simulink model "compare_model"  (R2022b)
settings: Solver=VariableStepAuto  StartTime=0.0  StopTime=t_samples*n_samples  RelTol=1e-3
values from neighbouring files (symbols this model uses):
  air_den = 1.225    [wind_turbine_parameters.m]
  l1 = 56    [wind_turbine_parameters.m]
  lambda_op = 5.68    [wind_turbine_parameters.m]
undefined symbols (not defined in the file or in its folder): pitch_deg, t_sample2
libraries: simulink x1, fuzblock x1
settings Model: Creator=luan  LastModifiedBy=marina

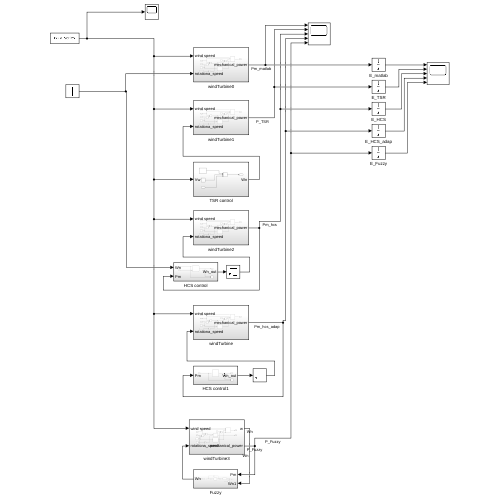
[thumbnail: Simulink's stored preview of the top-level diagram]
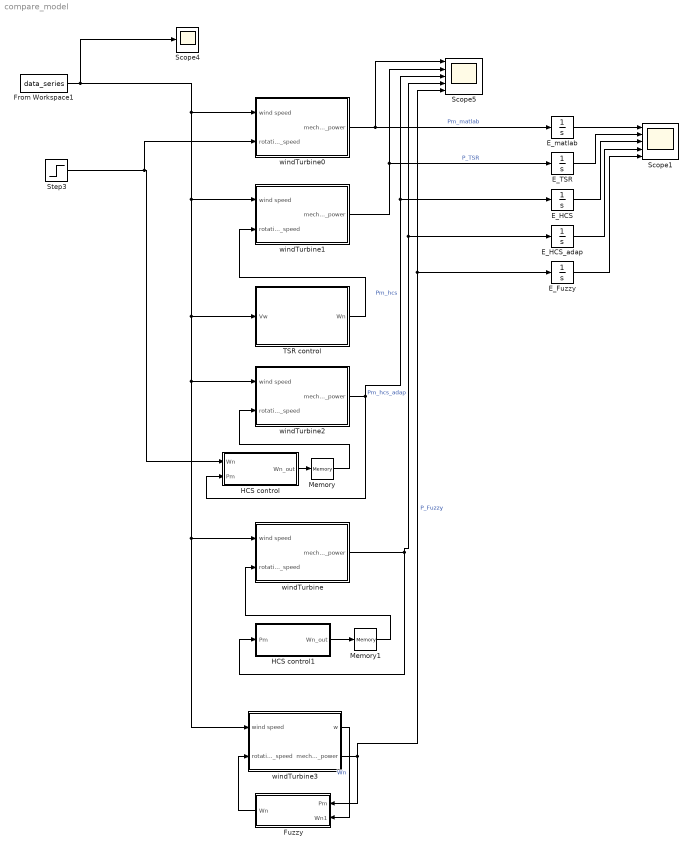
== system compare_model ==
  E_Fuzzy : Integrator
  E_HCS : Integrator
  E_HCS_adap : Integrator
  E_TSR : Integrator
  E_matlab : Integrator
  From Workspace1 : FromWorkspace  VariableName=data_series  SampleTime=t_sample2  OutputAfterFinalValue=Setting to zero
  Fuzzy : Subsystem
  HCS control : Subsystem
  HCS control1 : Subsystem
  Memory : Memory
  Memory1 : Memory
  Scope1 : Scope  NumInputPorts=5
  Scope4 : Scope
  Scope5 : Scope  NumInputPorts=5
  Step3 : Step  Time=0  After=0.9  SampleTime=0
  TSR control : Subsystem
  windTurbine : Subsystem
  windTurbine0 : Subsystem
  windTurbine1 : Subsystem
  windTurbine2 : Subsystem
  windTurbine3 : Subsystem
  wires:
  windTurbine0/1(mechanical_power) -> Scope5/1, E_matlab/1  "Pm_matlab"
  E_matlab/1 -> Scope1/1
  From Workspace1/1 -> Scope4/1, windTurbine0/1(wind speed), windTurbine1/1(wind speed), windTurbine2/1(wind speed), windTurbine3/1(wind speed), windTurbine/1(wind speed), TSR control/1(Vw)
  Step3/1 -> windTurbine0/2(rotationa_speed), HCS control/1(Wn)
  TSR control/1(Wn) -> windTurbine1/2(rotationa_speed)
  HCS control/1(Wn_out) -> Memory/1
  windTurbine2/1(mechanical_power) -> E_HCS/1, Scope5/3, HCS control/2(Pm)  "Pm_hcs"
  windTurbine/1(mechanical_power) -> E_HCS_adap/1, Scope5/4, HCS control1/1(Pm)  "Pm_hcs_adap"
  HCS control1/1(Wn_out) -> Memory1/1
  Memory1/1 -> windTurbine/2(rotationa_speed)
  windTurbine3/2(mechanical_power) -> E_Fuzzy/1, Scope5/5, Fuzzy/1(Pm)  "P_Fuzzy"
  windTurbine3/1(w) -> Fuzzy/2(Wn1)  "Wn"
  windTurbine1/1(mechanical_power) -> E_TSR/1, Scope5/2  "P_TSR"
  E_TSR/1 -> Scope1/2
  E_HCS_adap/1 -> Scope1/4
  E_HCS/1 -> Scope1/3
  E_Fuzzy/1 -> Scope1/5
  Memory/1 -> windTurbine2/2(rotationa_speed)
  Fuzzy/1(Wn) -> windTurbine3/2(rotationa_speed)

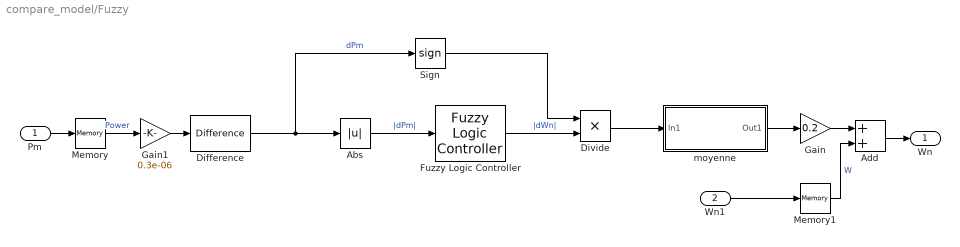
== system compare_model/Fuzzy ==
  Pm : Inport
  Wn1 : Inport  Port=2
  Abs : Abs  SaturateOnIntegerOverflow=off
  Add : Sum
  Difference : simulink/Discrete/Difference  ICPrevInput=0.0  OutMin=[]  OutMax=[]  OutDataType=fixdt(1, 16)  OutScaling=2^-10  DoSatur=off
  Divide : Product  Inputs=**
  Fuzzy Logic Controller : fuzblock/Fuzzy Logic  Controller  FIS='version1.fis'  OutputSampleNumber=101  DataType=double  FuzzifiedInputs=off  RuleFiringStrengths=off  RuleOutputs=off  AggregatedOutputs=off  SimulateUsing=Interpreted execution  OutOfRangeInputValueMessage=warning  NoRuleFiredMessage=warning  EmptyOutputFuzzySetMessage=warning
  Gain : Gain  Gain=0.2
  Gain1 : Gain  Gain=0.3e-06
  Memory : Memory
  Memory1 : Memory  InitialCondition=0.2
  Sign : Signum
  moyenne : Subsystem
  Wn : Outport
  wires:
  Abs/1 -> Fuzzy Logic Controller/1  "|dPm|"
  Add/1 -> Wn/1
  Difference/1 -> Sign/1, Abs/1  "dPm"
  Sign/1 -> Divide/1
  Fuzzy Logic Controller/1 -> Divide/2  "|dWn|"
  Divide/1 -> moyenne/1(In1)
  moyenne/1(Out1) -> Gain/1
  Gain/1 -> Add/1
  Gain1/1 -> Difference/1
  Memory1/1 -> Add/2  "W"
  Memory/1 -> Gain1/1  "Power"
  Pm/1 -> Memory/1
  Wn1/1 -> Memory1/1

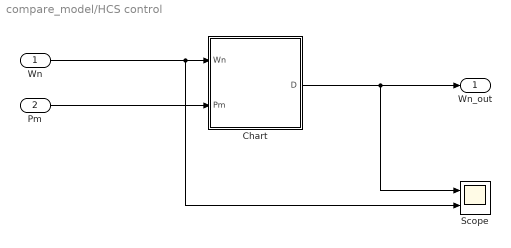
== system compare_model/HCS control ==
  Wn : Inport
  Pm : Inport  Port=2
  Chart : Stateflow chart  TreatAsAtomicUnit=on
  Scope : Scope  NumInputPorts=2
  Wn_out : Outport
  wires:
  Pm/1 -> Chart/2(Pm)
  Wn/1 -> Scope/2, Chart/1(Wn)
  Chart/1(D) -> Scope/1, Wn_out/1

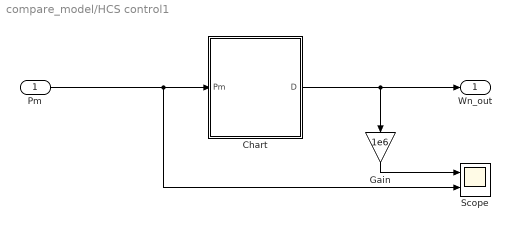
== system compare_model/HCS control1 ==
  Pm : Inport
  Chart : Stateflow chart  TreatAsAtomicUnit=on
  Gain : Gain  Gain=1e6
  Scope : Scope  NumInputPorts=2
  Wn_out : Outport
  wires:
  Chart/1(D) -> Gain/1, Wn_out/1
  Pm/1 -> Scope/2, Chart/1(Pm)
  Gain/1 -> Scope/1

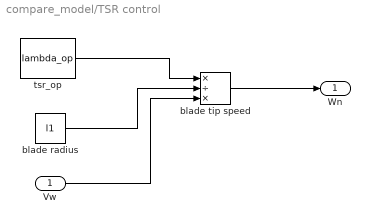
== system compare_model/TSR control ==
  Vw : Inport
  blade radius : Constant  Value=l1
  blade tip speed : Product  Inputs=*/*
  tsr_op : Constant  Value=lambda_op
  Wn : Outport
  wires:
  blade tip speed/1 -> Wn/1
  Vw/1 -> blade tip speed/3
  tsr_op/1 -> blade tip speed/1
  blade radius/1 -> blade tip speed/2

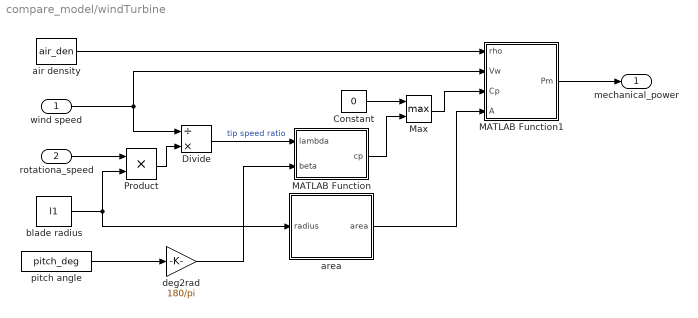
== system compare_model/windTurbine ==
  wind speed : Inport
  rotationa_speed : Inport  Port=2
  Constant : Constant  Value=0
  Divide : Product  Inputs=/*
  MATLAB Function : MATLAB Function  TreatAsAtomicUnit=on
  MATLAB Function1 : MATLAB Function  TreatAsAtomicUnit=on
  Max : MinMax  Function=max  Inputs=2
  Product : Product
  air density : Constant  Value=air_den
  area : Subsystem
  blade radius : Constant  Value=l1
  deg2rad : Gain  Gain=180/pi
  pitch angle : Constant  Value=pitch_deg
  mechanical_power : Outport
  wires:
  Product/1 -> Divide/2
  wind speed/1 -> Divide/1, MATLAB Function1/2(Vw)
  Divide/1 -> MATLAB Function/1(lambda)  "tip speed ratio"
  MATLAB Function1/1(Pm) -> mechanical_power/1
  rotationa_speed/1 -> Product/1
  air density/1 -> MATLAB Function1/1(rho)
  area/1(area) -> MATLAB Function1/4(A)
  blade radius/1 -> Product/2, area/1(radius)
  deg2rad/1 -> MATLAB Function/2(beta)
  Max/1 -> MATLAB Function1/3(Cp)
  MATLAB Function/1(cp) -> Max/2
  Constant/1 -> Max/1
  pitch angle/1 -> deg2rad/1

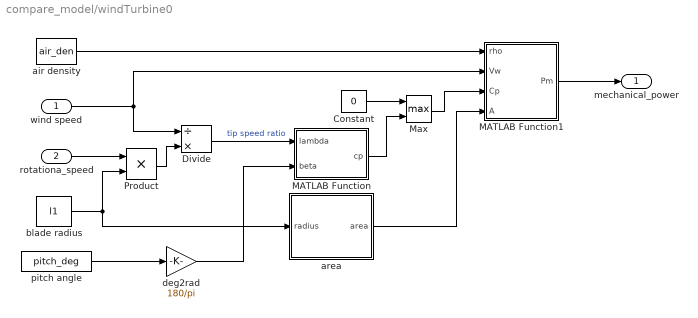
== system compare_model/windTurbine0 ==
  wind speed : Inport
  rotationa_speed : Inport  Port=2
  Constant : Constant  Value=0
  Divide : Product  Inputs=/*
  MATLAB Function : MATLAB Function  TreatAsAtomicUnit=on
  MATLAB Function1 : MATLAB Function  TreatAsAtomicUnit=on
  Max : MinMax  Function=max  Inputs=2
  Product : Product
  air density : Constant  Value=air_den
  area : Subsystem
  blade radius : Constant  Value=l1
  deg2rad : Gain  Gain=180/pi
  pitch angle : Constant  Value=pitch_deg
  mechanical_power : Outport
  wires:
  Product/1 -> Divide/2
  wind speed/1 -> Divide/1, MATLAB Function1/2(Vw)
  Divide/1 -> MATLAB Function/1(lambda)  "tip speed ratio"
  MATLAB Function1/1(Pm) -> mechanical_power/1
  rotationa_speed/1 -> Product/1
  air density/1 -> MATLAB Function1/1(rho)
  area/1(area) -> MATLAB Function1/4(A)
  blade radius/1 -> Product/2, area/1(radius)
  deg2rad/1 -> MATLAB Function/2(beta)
  Max/1 -> MATLAB Function1/3(Cp)
  MATLAB Function/1(cp) -> Max/2
  Constant/1 -> Max/1
  pitch angle/1 -> deg2rad/1

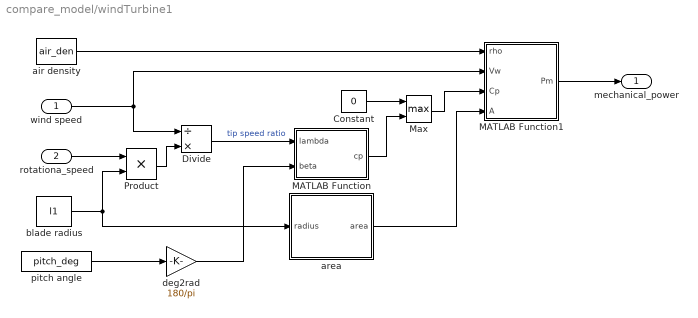
== system compare_model/windTurbine1 ==
  wind speed : Inport
  rotationa_speed : Inport  Port=2
  Constant : Constant  Value=0
  Divide : Product  Inputs=/*
  MATLAB Function : MATLAB Function  TreatAsAtomicUnit=on
  MATLAB Function1 : MATLAB Function  TreatAsAtomicUnit=on
  Max : MinMax  Function=max  Inputs=2
  Product : Product
  air density : Constant  Value=air_den
  area : Subsystem
  blade radius : Constant  Value=l1
  deg2rad : Gain  Gain=180/pi
  pitch angle : Constant  Value=pitch_deg
  mechanical_power : Outport
  wires:
  Product/1 -> Divide/2
  wind speed/1 -> Divide/1, MATLAB Function1/2(Vw)
  Divide/1 -> MATLAB Function/1(lambda)  "tip speed ratio"
  MATLAB Function1/1(Pm) -> mechanical_power/1
  rotationa_speed/1 -> Product/1
  air density/1 -> MATLAB Function1/1(rho)
  area/1(area) -> MATLAB Function1/4(A)
  blade radius/1 -> Product/2, area/1(radius)
  deg2rad/1 -> MATLAB Function/2(beta)
  Max/1 -> MATLAB Function1/3(Cp)
  MATLAB Function/1(cp) -> Max/2
  Constant/1 -> Max/1
  pitch angle/1 -> deg2rad/1

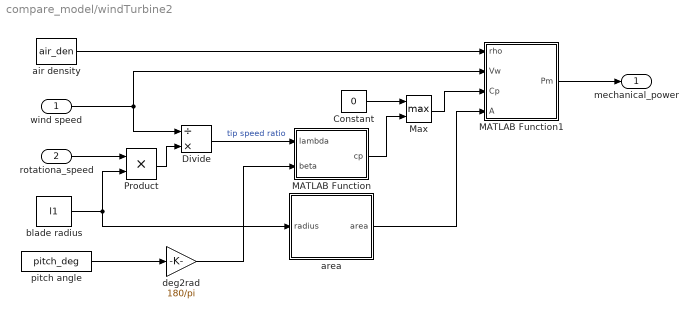
== system compare_model/windTurbine2 ==
  wind speed : Inport
  rotationa_speed : Inport  Port=2
  Constant : Constant  Value=0
  Divide : Product  Inputs=/*
  MATLAB Function : MATLAB Function  TreatAsAtomicUnit=on
  MATLAB Function1 : MATLAB Function  TreatAsAtomicUnit=on
  Max : MinMax  Function=max  Inputs=2
  Product : Product
  air density : Constant  Value=air_den
  area : Subsystem
  blade radius : Constant  Value=l1
  deg2rad : Gain  Gain=180/pi
  pitch angle : Constant  Value=pitch_deg
  mechanical_power : Outport
  wires:
  Product/1 -> Divide/2
  wind speed/1 -> Divide/1, MATLAB Function1/2(Vw)
  Divide/1 -> MATLAB Function/1(lambda)  "tip speed ratio"
  MATLAB Function1/1(Pm) -> mechanical_power/1
  rotationa_speed/1 -> Product/1
  air density/1 -> MATLAB Function1/1(rho)
  area/1(area) -> MATLAB Function1/4(A)
  blade radius/1 -> Product/2, area/1(radius)
  deg2rad/1 -> MATLAB Function/2(beta)
  Max/1 -> MATLAB Function1/3(Cp)
  MATLAB Function/1(cp) -> Max/2
  Constant/1 -> Max/1
  pitch angle/1 -> deg2rad/1

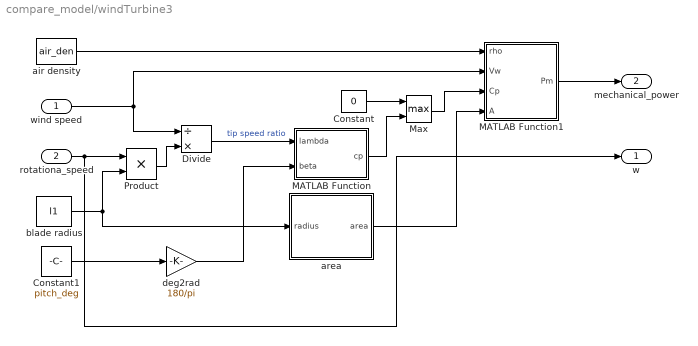
== system compare_model/windTurbine3 ==
  wind speed : Inport
  rotationa_speed : Inport  Port=2
  Constant : Constant  Value=0
  Constant1 : Constant  Value=pitch_deg
  Divide : Product  Inputs=/*
  MATLAB Function : MATLAB Function  TreatAsAtomicUnit=on
  MATLAB Function1 : MATLAB Function  TreatAsAtomicUnit=on
  Max : MinMax  Function=max  Inputs=2
  Product : Product
  air density : Constant  Value=air_den
  area : Subsystem
  blade radius : Constant  Value=l1
  deg2rad : Gain  Gain=180/pi
  w : Outport
  mechanical_power : Outport  Port=2
  wires:
  Product/1 -> Divide/2
  wind speed/1 -> Divide/1, MATLAB Function1/2(Vw)
  Divide/1 -> MATLAB Function/1(lambda)  "tip speed ratio"
  Constant1/1 -> deg2rad/1
  MATLAB Function1/1(Pm) -> mechanical_power/1
  rotationa_speed/1 -> w/1, Product/1
  air density/1 -> MATLAB Function1/1(rho)
  area/1(area) -> MATLAB Function1/4(A)
  blade radius/1 -> Product/2, area/1(radius)
  deg2rad/1 -> MATLAB Function/2(beta)
  Max/1 -> MATLAB Function1/3(Cp)
  MATLAB Function/1(cp) -> Max/2
  Constant/1 -> Max/1

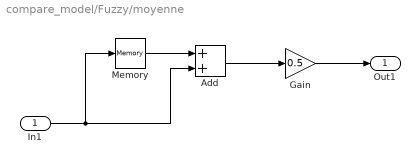
== system compare_model/Fuzzy/moyenne ==
  In1 : Inport
  Add : Sum
  Gain : Gain  Gain=0.5
  Memory : Memory
  Out1 : Outport
  wires:
  In1/1 -> Memory/1, Add/2
  Memory/1 -> Add/1
  Add/1 -> Gain/1
  Gain/1 -> Out1/1

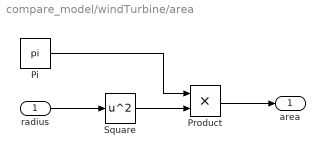
== system compare_model/windTurbine/area ==
  radius : Inport
  Pi : Constant  Value=pi  OutDataTypeStr=Inherit: Inherit via back propagation
  Product : Product
  Square : Math  Operator=square
  area : Outport
  wires:
  radius/1 -> Square/1
  Square/1 -> Product/2
  Pi/1 -> Product/1
  Product/1 -> area/1

== system compare_model/windTurbine0/area ==
  radius : Inport
  Pi : Constant  Value=pi  OutDataTypeStr=Inherit: Inherit via back propagation
  Product : Product
  Square : Math  Operator=square
  area : Outport
  wires:
  radius/1 -> Square/1
  Square/1 -> Product/2
  Pi/1 -> Product/1
  Product/1 -> area/1

== system compare_model/windTurbine1/area ==
  radius : Inport
  Pi : Constant  Value=pi  OutDataTypeStr=Inherit: Inherit via back propagation
  Product : Product
  Square : Math  Operator=square
  area : Outport
  wires:
  radius/1 -> Square/1
  Square/1 -> Product/2
  Pi/1 -> Product/1
  Product/1 -> area/1

== system compare_model/windTurbine2/area ==
  radius : Inport
  Pi : Constant  Value=pi  OutDataTypeStr=Inherit: Inherit via back propagation
  Product : Product
  Square : Math  Operator=square
  area : Outport
  wires:
  radius/1 -> Square/1
  Square/1 -> Product/2
  Pi/1 -> Product/1
  Product/1 -> area/1

== system compare_model/windTurbine3/area ==
  radius : Inport
  Pi : Constant  Value=pi  OutDataTypeStr=Inherit: Inherit via back propagation
  Product : Product
  Square : Math  Operator=square
  area : Outport
  wires:
  radius/1 -> Square/1
  Square/1 -> Product/2
  Pi/1 -> Product/1
  Product/1 -> area/1

== matlab function compare_model/windTurbine1/MATLAB Function ==
  data: lambda input; cp output; beta input
function cp = fcn(lambda, beta)

k = load('coefficients.mat');
lambda_i =  1/(1/(lambda + 0.08*beta) - 0.035/(1+beta*beta*beta));

% Debug
% lambda_i
% k.k1 *(k.k2/lambda_i - k.k3*beta - k.k4*power(beta, k.k5) -k.k6)*exp(-k.k7/lambda_i)

cp = k.k1 *(k.k2/lambda_i - k.k3*beta - k.k4*power(beta, k.k5) -k.k6)*exp(-k.k7/lambda_i);

== matlab function compare_model/windTurbine1/MATLAB Function1 ==
  data: rho input; Vw input; Pm output; Cp input; A input
function Pm = fcn(rho, Vw, Cp, A)

Pm = 0.5* Cp* rho* A* power(Vw, 3);

== matlab function compare_model/windTurbine0/MATLAB Function ==
  data: lambda input; cp output; beta input
function cp = fcn(lambda, beta)

k = load('coefficients.mat');
lambda_i =  1/(1/(lambda + 0.08*beta) - 0.035/(1+beta*beta*beta));

% Debug
% lambda_i
% k.k1 *(k.k2/lambda_i - k.k3*beta - k.k4*power(beta, k.k5) -k.k6)*exp(-k.k7/lambda_i)

cp = k.k1 *(k.k2/lambda_i - k.k3*beta - k.k4*power(beta, k.k5) -k.k6)*exp(-k.k7/lambda_i);

== matlab function compare_model/windTurbine0/MATLAB Function1 ==
  data: rho input; Vw input; Pm output; Cp input; A input
function Pm = fcn(rho, Vw, Cp, A)

Pm = 0.5* Cp* rho* A* power(Vw, 3);

== stateflow chart compare_model/HCS control/Chart ==
  state stationary
    entry:
    D = Wn;
  state init_
    entry:
    D = Wn;
    pt_1 = 0;
    d_ = d;
  state measure
    entry:
    dp = Pm - pt_1;
    pt_1 = Pm;
  state decrease
    entry:
    d_ = - d_;
  state increase
    entry:
    d_ = d_;
  state perturb_
    entry:
    D = D + d_;
  measure -> stationary [order 3] : [abs(dp)< 500]
  stationary -> measure : [after(delay,sec)]
  (default) -> init_
  measure -> decrease [order 2] : [dp < 0]
  init_ -> measure
  perturb_ -> measure : [after(delay,sec)]
  decrease -> perturb_
  measure -> increase [order 1] : [dp > 0]
  increase -> perturb_
  data: Wn input; Pm input; D output; delay constant double =5; d constant double =0.05; pt_1 local; dp local; d_ local

== matlab function compare_model/windTurbine2/MATLAB Function ==
  data: lambda input; cp output; beta input
function cp = fcn(lambda, beta)

k = load('coefficients.mat');
lambda_i =  1/(1/(lambda + 0.08*beta) - 0.035/(1+beta*beta*beta));

% Debug
% lambda_i
% k.k1 *(k.k2/lambda_i - k.k3*beta - k.k4*power(beta, k.k5) -k.k6)*exp(-k.k7/lambda_i)

cp = k.k1 *(k.k2/lambda_i - k.k3*beta - k.k4*power(beta, k.k5) -k.k6)*exp(-k.k7/lambda_i);

== matlab function compare_model/windTurbine2/MATLAB Function1 ==
  data: rho input; Vw input; Pm output; Cp input; A input
function Pm = fcn(rho, Vw, Cp, A)

Pm = 0.5* Cp* rho* A* power(Vw, 3);

== stateflow chart compare_model/HCS control1/Chart ==
  state init_
    entry:
    D = 1;
    pt_1 = Pm;
    direction = 1;
  state perturb_
    entry:
    D = D + d_;
    D = max(D, 0);
    pt_1 = Pm;
  state measure
    entry:
    dp = Pm - pt_1;
  state keep_direction
    entry:
    direction = direction;
  state update
    entry:
    d_ = direction * Gamma * abs(dp);
  state change_direction
    entry:
    direction = -1* direction;
  state perturb
    entry:
    d_ = randn(1)/500;
    direction = d_/abs(d_);
  (junction 73) -> (junction 74)
  (default) -> init_
  (junction 74) -> measure
  (junction 77) -> (junction 73)
  update -> perturb_
  init_ -> measure
  measure -> keep_direction [order 2] : [dp > Tr]
  keep_direction -> update
  perturb_ -> (junction 77) : [after(delay,sec)]
  (junction 99) -> update
  measure -> perturb [order 3]
  measure -> (junction 95) [order 1] : [dp < -Tr]
  (junction 121) -> perturb_
  (junction 95) -> change_direction
  change_direction -> (junction 99)
  perturb -> (junction 121)
  data: Pm input; D output; delay constant double =30; pt_1 local =1000; dp local; Gamma constant double =1e-7; d_ local; direction local; Tr constant double

== matlab function compare_model/windTurbine/MATLAB Function ==
  data: lambda input; cp output; beta input
function cp = fcn(lambda, beta)

k = load('coefficients.mat');
lambda_i =  1/(1/(lambda + 0.08*beta) - 0.035/(1+beta*beta*beta));

% Debug
% lambda_i
% k.k1 *(k.k2/lambda_i - k.k3*beta - k.k4*power(beta, k.k5) -k.k6)*exp(-k.k7/lambda_i)

cp = k.k1 *(k.k2/lambda_i - k.k3*beta - k.k4*power(beta, k.k5) -k.k6)*exp(-k.k7/lambda_i);

== matlab function compare_model/windTurbine/MATLAB Function1 ==
  data: rho input; Vw input; Pm output; Cp input; A input
function Pm = fcn(rho, Vw, Cp, A)

Pm = 0.5* Cp* rho* A* power(Vw, 3);

== matlab function compare_model/windTurbine3/MATLAB Function ==
  data: lambda input; cp output; beta input
function cp = fcn(lambda, beta)

k = load('coefficients.mat');
lambda_i =  1/(1/(lambda + 0.08*beta) - 0.035/(1+beta*beta*beta));

% Debug
% lambda_i
% k.k1 *(k.k2/lambda_i - k.k3*beta - k.k4*power(beta, k.k5) -k.k6)*exp(-k.k7/lambda_i)

cp = k.k1 *(k.k2/lambda_i - k.k3*beta - k.k4*power(beta, k.k5) -k.k6)*exp(-k.k7/lambda_i);

== matlab function compare_model/windTurbine3/MATLAB Function1 ==
  data: rho input; Vw input; Pm output; Cp input; A input
function Pm = fcn(rho, Vw, Cp, A)

Pm = 0.5* Cp* rho* A* power(Vw, 3);
